simulink model "compensated_buckboost"  (R2021a)
settings: Solver=VariableStepAuto  StartTime=0.0  StopTime=0.05  RelTol=1e-3
values from neighbouring files (symbols this model uses):
  C = 220e-6    (= 0.00022)    [buckboost_compensator.m]    (also in buckboost_tfs.m = 0.00016)
  H = 1/(1+s/wf)    [boost_tfs.m]    (also in buckboost_compensator.m = -0.333333333333)
  L = 50e-6    (= 5e-05)    [buckboost_compensator.m]    (also in buckboost_tfs.m = 0.00016)
  R = V/Iout    (= 245)    [boost_tfs.m]    (also in buckboost_compensator.m = 5; buckboost_tfs.m = 10)
  Vg = 170    [boost_tfs.m]    (also in buckboost_compensator.m = 48; buckboost_tfs.m = 30)
  Vm = 2    [boost_tfs.m]    (also in buckboost_compensator.m = 3)
  Vref = 5    [buckboost_compensator.m]
libraries: spsControlledVoltageSourceLib x3, spsGroundLib x3, spsControlledCurrentSourceLib x2, spsSeriesRLCBranchLib x2, spsVoltageMeasurementLib x2, spsCurrentMeasurementLib x1, spsIdealSwitchLib x1, cstblocks x1, spspowerguiLib x1
settings Model: Creator=jneat  LastModifiedBy=jneat

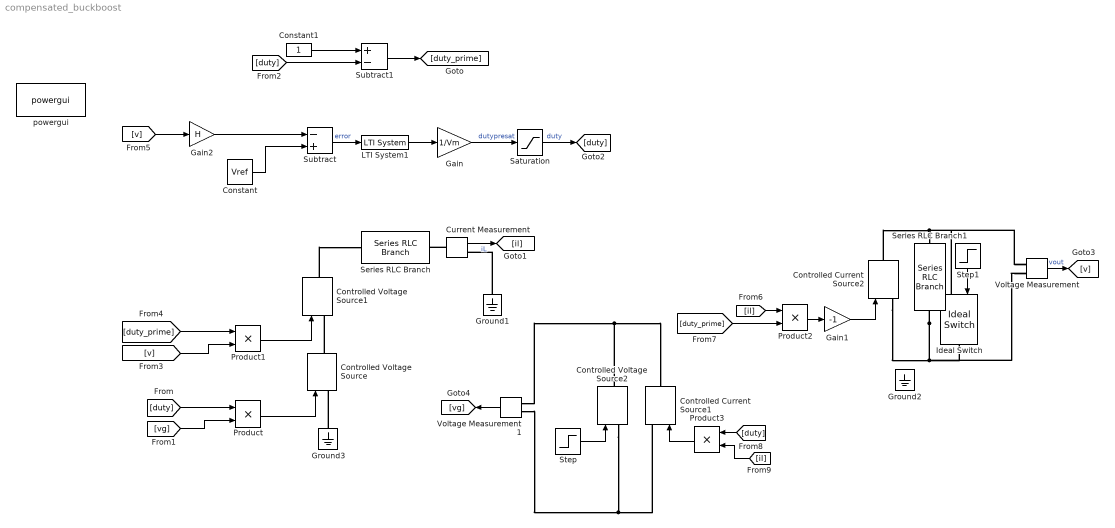
== system compensated_buckboost ==
  Constant : Constant  Value=Vref
  Constant1 : Constant
  Controlled Current Source1 : spsControlledCurrentSourceLib/Controlled Current Source  Initialize=on  Source_Type=AC  Amplitude=0  Phase=0  Frequency=0  Measurements=None
  Controlled Current Source2 : spsControlledCurrentSourceLib/Controlled Current Source  Initialize=on  Source_Type=AC  Amplitude=0  Phase=0  Frequency=0  Measurements=None
  Controlled Voltage Source : spsControlledVoltageSourceLib/Controlled Voltage Source  Initialize=on  Source_Type=AC  Amplitude=0  Phase=0  Frequency=0  Measurements=None
  Controlled Voltage Source1 : spsControlledVoltageSourceLib/Controlled Voltage Source  Initialize=on  Source_Type=AC  Amplitude=0  Phase=0  Frequency=0  Measurements=None
  Controlled Voltage Source2 : spsControlledVoltageSourceLib/Controlled Voltage Source  Initialize=on  Source_Type=AC  Amplitude=0  Phase=0  Frequency=0  Measurements=None
  Current Measurement : spsCurrentMeasurementLib/Current Measurement  PhasorSimulation=off  OutputType=Complex  PSBequivalent=0
  Gain : Gain  Gain=1/Vm
  Gain1 : Gain  Gain=-1
  Gain2 : Gain  Gain=H
  Ground1 : spsGroundLib/Ground  LConnTagsString=a
  Ground2 : spsGroundLib/Ground  LConnTagsString=a
  Ground3 : spsGroundLib/Ground  LConnTagsString=a
  Ideal Switch : spsIdealSwitchLib/Ideal Switch  Ron=R/2  Lon=0  IC=0  Rs=R  Cs=inf  Measurements=off
  LTI System1 : cstblocks/LTI System  sys=Gc  IC=[]
  Product{,1..3} (4 alike) : Product
  Saturation : Saturate  UpperLimit=1  LowerLimit=0
  Series RLC Branch : spsSeriesRLCBranchLib/Series RLC Branch  LConnTagsString=__new0  RConnTagsString=__new0  BranchType=L  Resistance=1  Inductance=L  SetiL0=off  InitialCurrent=0  Capacitance=1e-6  Setx0=off  InitialVoltage=0  Measurements=None
  Series RLC Branch1 : spsSeriesRLCBranchLib/Series RLC Branch  LConnTagsString=__new0  RConnTagsString=__new0  BranchType=C  Resistance=1  Inductance=1e-3  SetiL0=off  InitialCurrent=0  Capacitance=C  Setx0=on  InitialVoltage=-10  Measurements=None
  Step : Step  Time=0  Before=Vg  After=Vg  SampleTime=0
  Step1 : Step  Time=0.03  SampleTime=0
  Subtract : Sum  Inputs=-+
  Subtract1 : Sum  Inputs=+-
  Voltage Measurement : spsVoltageMeasurementLib/Voltage Measurement  PhasorSimulation=off  OutputType=Complex  PSBequivalent=0
  Voltage Measurement1 : spsVoltageMeasurementLib/Voltage Measurement  PhasorSimulation=off  OutputType=Complex  PSBequivalent=0
  powergui : spspowerguiLib/powergui  Priority=1  SimulationMode=Continuous  SampleTime=50e-6  frequency=60  Iterations=50  frequencyindice=0  Pbase=100e6  ErrMax=1e-4  UnitsV=kV  UnitsW=MW  buscounter=0  FunctionMessages=off  echomessages=off  EnableUseOfTLC=off  CurrentSourceSwitches=off  DisableSnubberDevices=off  DisableRonSwitches=off  DisableVfSwitches=off  DisplayEquations=off  AutomaticDiscreteSolvers=off  SolverType=Tustin/Backward Euler (TBE)  Interpol=off  ExternalGateDelay=off  methode=off  Ts=100  x0status=blocks  SPID=on  SwTol=0  HookPort=off  NonlinearTolerance=1e-4  nMaxIteration=100  ContinueOnMaxIteration=off  RestoreLinks=warning  ResistiveCurrentMeasurement=off  Frange=[0:2:500]  Ylog=off  Xlog=on  ShowGrid=off  save=off  variable=ZData  structure=0  ZoomFFT=off  StartTime=0.0  cycles=1  DisplayStyle=1  fundamental=60  FreqAxis=off  MaxFrequency=1000  frequencyindicesteady=1  RmsSteady=1  display=off
  wires:
  Subtract/1 -> LTI System1/1  "error"
  LTI System1/1 -> Gain/1
  Gain/1 -> Saturation/1  "dutypresat"
  Gain2/1 -> Subtract/1
  Constant/1 -> Subtract/2
  Product/1 -> Controlled Voltage Source/1
  Product1/1 -> Controlled Voltage Source1/1
  Constant1/1 -> Subtract1/1
  [duty] -> Subtract1/2
  Subtract1/1 -> [duty_prime]
  [duty_prime] -> Product1/1
  [v] -> Product1/2
  [duty] -> Product/1
  [vg] -> Product/2
  Current Measurement/1 -> [il]  "iL"
  Saturation/1 -> [duty]  "duty"
  [il] -> Product2/1
  [duty_prime] -> Product2/2
  Voltage Measurement/1 -> [v]  "vout"
  [duty] -> Product3/1
  [il] -> Product3/2
  Voltage Measurement1/1 -> [vg]
  Product3/1 -> Controlled Current Source1/1
  [v] -> Gain2/1
  Product2/1 -> Gain1/1
  Gain1/1 -> Controlled Current Source2/1
  Step/1 -> Controlled Voltage Source2/1
  Step1/1 -> Ideal Switch/1
  connections:
  Controlled Voltage Source/RConn1 -- Controlled Voltage Source1/LConn1
  Ground3/LConn1 -- Controlled Voltage Source/LConn1
  Controlled Voltage Source1/RConn1 -- Series RLC Branch/LConn1
  Ground1/LConn1 -- Current Measurement/RConn1
  Current Measurement/LConn1 -- Series RLC Branch/RConn1
  Voltage Measurement1/LConn1 -- Controlled Voltage Source2/RConn1 -- Controlled Current Source1/RConn1
  Voltage Measurement1/LConn2 -- Controlled Voltage Source2/LConn1 -- Controlled Current Source1/LConn1
  Controlled Current Source2/RConn1 -- Ideal Switch/LConn1 -- Voltage Measurement/LConn1 -- Series RLC Branch1/LConn1
  Series RLC Branch1/RConn1 -- Ideal Switch/RConn1 -- Voltage Measurement/LConn2 -- Controlled Current Source2/LConn1
